simulink model "pc_mdl"  (Simulink 4.00)
settings: Solver=ode45  StartTime=0.0  StopTime=10.0  RelTol=1e-3
settings Model: BlockReductionOpt=off

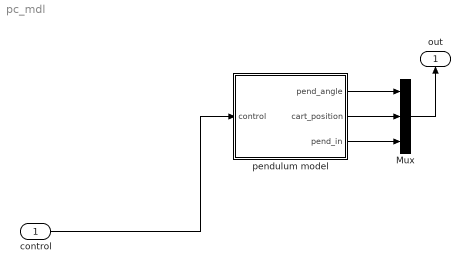
== system pc_mdl ==
  control : Inport  Port=1
  Mux : Mux  Inputs=3
  pendulum model : Subsystem  mask{cmass=0.5, cfriction=0.05, mass=.275, length=0.5, friction=0.01, Tmax=10, quant=.001, stiction=.001, IC=180}
      mask prompts: cmass "cart mass"; cfriction "cart friction coeff"; mass "pendulum mass"; length "pendulum length"; friction "pendulum friction coeff"; Tmax "Max force"; quant "quantization (deg)"; stiction "stiction dead-zone (rad/s)"; IC "Initial condition (deg, 0 velocity)"
      settings: RTWFcnNameOpts=Auto  RTWFileNameOpts=Auto
  out : Outport  Orientation=up  Port=1  InitialOutput=0
  wires:
  pendulum model/1(pend_angle) -> Mux/1
  pendulum model/2(cart_position) -> Mux/2
  Mux/1 -> out/1
  pendulum model/3(pend_in) -> Mux/3
  control/1 -> pendulum model/1(control)

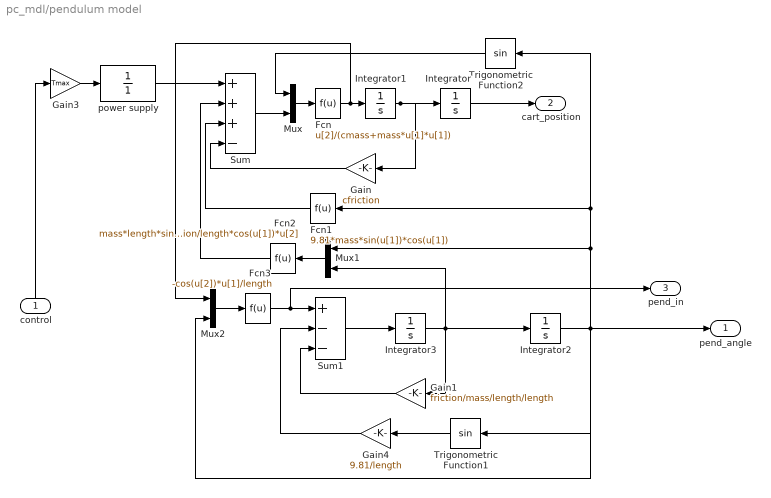
== system pc_mdl/pendulum model ==
  control : Inport  Orientation=up  Port=1
  Fcn : Fcn  Expr=u[2]/(cmass+mass*u[1]*u[1])
  Fcn1 : Fcn  Orientation=left  Expr=9.81*mass*sin(u[1])*cos(u[1])
  Fcn2 : Fcn  Orientation=left  Expr=mass*length*sin(u[1])*u[2]*u[2]+friction/length*cos(u[1])*u[2]
  Fcn3 : Fcn  Expr=-cos(u[2])*u[1]/length
  Gain : Gain  Orientation=left  Gain=cfriction  Multiplication=Element-wise(K.*u)  SaturateOnIntegerOverflow=on
  Gain1 : Gain  Orientation=left  Gain=friction/mass/length/length  Multiplication=Element-wise(K.*u)  SaturateOnIntegerOverflow=on
  Gain3 : Gain  Gain=Tmax  Multiplication=Element-wise(K.*u)  SaturateOnIntegerOverflow=on
  Gain4 : Gain  Orientation=left  Gain=9.81/length  Multiplication=Element-wise(K.*u)  SaturateOnIntegerOverflow=on
  Integrator : Integrator  ExternalReset=none  InitialConditionSource=internal  InitialCondition=0  LimitOutput=off  UpperSaturationLimit=inf  LowerSaturationLimit=-inf  ShowSaturationPort=off  ShowStatePort=off  AbsoluteTolerance=auto
  Integrator1 : Integrator  ExternalReset=none  InitialConditionSource=internal  InitialCondition=0  LimitOutput=off  UpperSaturationLimit=inf  LowerSaturationLimit=-inf  ShowSaturationPort=off  ShowStatePort=off  AbsoluteTolerance=auto
  Integrator2 : Integrator  ExternalReset=none  InitialConditionSource=internal  InitialCondition=IC*pi/180  LimitOutput=off  UpperSaturationLimit=inf  LowerSaturationLimit=-inf  ShowSaturationPort=off  ShowStatePort=off  AbsoluteTolerance=auto
  Integrator3 : Integrator  ExternalReset=none  InitialConditionSource=internal  InitialCondition=0  LimitOutput=off  UpperSaturationLimit=inf  LowerSaturationLimit=-inf  ShowSaturationPort=off  ShowStatePort=off  AbsoluteTolerance=auto
  Mux : Mux  Inputs=2
  Mux1 : Mux  Orientation=left  Inputs=2
  Mux2 : Mux  Inputs=2
  Sum : Sum  Inputs=+++-  SaturateOnIntegerOverflow=on
  Sum1 : Sum  Inputs=+--  SaturateOnIntegerOverflow=on
  Trigonometric Function1 : Trigonometry  Orientation=left  Operator=sin  OutputSignalType=auto
  Trigonometric Function2 : Trigonometry  Orientation=left  Operator=sin  OutputSignalType=auto
  power supply : TransferFcn  Numerator=1  Denominator=1  Realization=auto  AbsoluteTolerance=auto
  pend_angle : Outport  Port=1  InitialOutput=0
  cart_position : Outport  Port=2  InitialOutput=0
  pend_in : Outport  Port=3  InitialOutput=0
  wires:
  Integrator1/1 -> Gain/1, Integrator/1
  Integrator/1 -> cart_position/1
  Gain3/1 -> power supply/1
  power supply/1 -> Sum/1
  control/1 -> Gain3/1
  Sum1/1 -> Integrator3/1
  Integrator3/1 -> Gain1/1, Mux1/2, Integrator2/1
  Gain1/1 -> Sum1/3
  Integrator2/1 -> Trigonometric Function1/1, Mux1/1, Fcn1/1, Trigonometric Function2/1, Mux2/2, pend_angle/1
  Trigonometric Function1/1 -> Gain4/1
  Gain4/1 -> Sum1/2
  Fcn/1 -> Integrator1/1, Mux2/1
  Mux/1 -> Fcn/1
  Sum/1 -> Mux/2
  Gain/1 -> Sum/4
  Fcn1/1 -> Sum/3
  Mux1/1 -> Fcn2/1
  Fcn2/1 -> Sum/2
  Fcn3/1 -> Sum1/1, pend_in/1
  Mux2/1 -> Fcn3/1
  Trigonometric Function2/1 -> Mux/1
